simulink model "Simu_Simulink"  (R2016a)
settings: Solver=FixedStepDiscrete  StartTime=0.0  StopTime=50  FixedStep=0.01  RelTol=1e-3
values from neighbouring files (symbols this model uses):
  lambdaSplit = reshape(lambda,lambdaDim,sizeSeg,DoP)    [Simu_Matlab.m]    (also in Simu_Matlab_test.m = lambdaSplitNew; Simu_Simulink_Setup.m = reshape(lambda, lambdaDim,  sizeSeg,DoP))
  LAMBDASplit = reshape(LAMBDA,xDim,xDim,sizeSeg,DoP)    [Simu_Matlab.m]    (also in Simu_Matlab_test.m; Simu_Simulink_Setup.m = reshape(LAMBDA, xDim, xDim, sizeSeg,DoP))
  pSplit = reshape(par,pDim,sizeSeg,DoP)    [Simu_Matlab.m]    (also in Simu_Matlab_test.m; Simu_Simulink_Setup.m = reshape(par,    pDim,       sizeSeg,DoP))
  uSplit = reshape(u,uDim,sizeSeg,DoP)    [Simu_Matlab.m]    (also in Simu_Matlab_test.m; Simu_Simulink_Setup.m = reshape(u,      uDim,       sizeSeg,DoP))
  x0 = [1 0 1 0 1 0 0 0 0]    [GEN_initData.mat]    (also in NMPC_Problem_Formulation.m = [1;0;1;0;1;0;0;0;0]; Simu_Matlab.m = SIM_Plant_RK4(uOpt(1:4,1),x0,pSimVal,Ts); Simu_Matlab_test.m = SIM_Plant_RK4(uOpt(1:4,1),x0,pSimVal,Ts); Simu_Simulink_Setup.m = data.x0)
  xSplit = reshape(x,xDim,sizeSeg,DoP)    [Simu_Matlab.m]    (also in Simu_Matlab_test.m = xSplitNew; Simu_Simulink_Setup.m = reshape(x,      xDim,       sizeSeg,DoP))
settings Model: Creator=Deng  LastModifiedBy=Deng
settings OptimizationCC: SimCompilerOptimization=on
settings HardwareCC: ProdWordSize=32  ProdHWDeviceType=Specified
settings SFSimCC: SimCustomHeaderCode="#include \"NMPC_Iter.h\""  SimUserLibraries=NMPC_Iter.lib
settings SFSimCC: SimUserIncludeDirs=|
  | ./codegen/dll/NMPC_Iter
  | ./codegen/lib/OCP_F_Fu_Fx
settings RTWCC: GenerateReport=on  RTWUseSimCustomCode=on  CustomHeaderCode="#include \"NMPC_Iter.h\""  CustomLibrary=NMPC_Iter.lib  BuildConfiguration=Faster Runs  LaunchReport=on
settings RTWCC: CustomInclude=|
  | ./codegen/dll/NMPC_Iter
  | ./codegen/lib/OCP_F_Fu_Fx

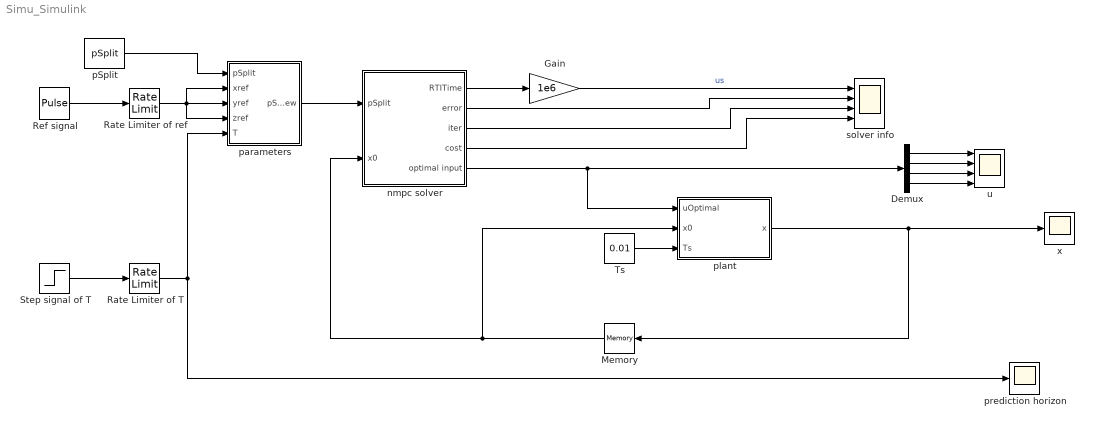
== system Simu_Simulink ==
  Demux : Demux
  Gain : Gain  Gain=1e6
  Memory : Memory  X0=x0
  Rate Limiter of T : RateLimiter  SampleTimeMode=inherited
  Rate Limiter of ref : RateLimiter  RisingSlewLimit=10  SampleTimeMode=inherited
  Ref signal : DiscretePulseGenerator  PulseType=Time based  Period=20  PulseWidth=50  PhaseDelay=10
  Step signal of T : Step  Time=25  Before=1  After=0.5  SampleTime=0
  Ts : Constant  Value=0.01
  nmpc solver : Subsystem
  pSplit : Constant  Value=pSplit
  parameters : MATLAB Function  TreatAsAtomicUnit=on
  plant : MATLAB Function  TreatAsAtomicUnit=on
  prediction horizon : Scope
  solver info : Scope  NumInputPorts=4
  u : Scope  NumInputPorts=4
  x : Scope
  wires:
  Memory/1 -> nmpc solver/2(x0), plant/2(x0)
  plant/1(x) -> Memory/1, x/1
  Ts/1 -> plant/3(Ts)
  pSplit/1 -> parameters/1(pSplit)
  Rate Limiter of ref/1 -> parameters/2(xref), parameters/4(zref), parameters/3(yref)
  parameters/1(pSplitNew) -> nmpc solver/1(pSplit)
  nmpc solver/5(optimal input) -> plant/1(uOptimal), Demux/1
  Demux/1 -> u/1
  Demux/2 -> u/2
  Demux/3 -> u/3
  Demux/4 -> u/4
  nmpc solver/2(error) -> solver info/2
  nmpc solver/1(RTITime) -> Gain/1
  nmpc solver/4(cost) -> solver info/4
  Ref signal/1 -> Rate Limiter of ref/1
  nmpc solver/3(iter) -> solver info/3
  Gain/1 -> solver info/1  "us"
  Step signal of T/1 -> Rate Limiter of T/1
  Rate Limiter of T/1 -> prediction horizon/1, parameters/5(T)

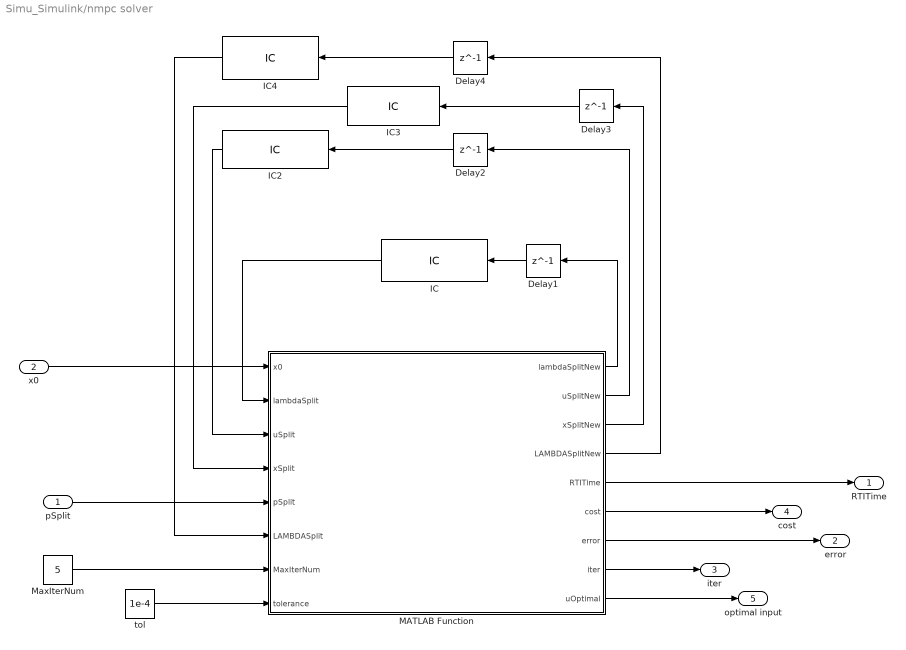
== system Simu_Simulink/nmpc solver ==
  pSplit : Inport
  x0 : Inport  Port=2
  Delay{1..4} (4 alike) : Delay  DelayLength=1  InitialCondition=0
  IC : InitialCondition  Value=lambdaSplit
  IC2 : InitialCondition  Value=uSplit
  IC3 : InitialCondition  Value=xSplit
  IC4 : InitialCondition  Value=LAMBDASplit
  MATLAB Function : MATLAB Function  TreatAsAtomicUnit=on
  MaxIterNum : Constant  Value=5
  tol : Constant  Value=1e-4
  RTITime : Outport
  error : Outport  Port=2
  iter : Outport  Port=3
  cost : Outport  Port=4
  optimal input : Outport  Port=5
  wires:
  Delay2/1 -> IC2/1
  Delay1/1 -> IC/1
  Delay4/1 -> IC4/1
  Delay3/1 -> IC3/1
  MaxIterNum/1 -> MATLAB Function/7(MaxIterNum)
  tol/1 -> MATLAB Function/8(tolerance)
  MATLAB Function/5(RTITime) -> RTITime/1
  MATLAB Function/6(cost) -> cost/1
  MATLAB Function/7(error) -> error/1
  MATLAB Function/9(uOptimal) -> optimal input/1
  x0/1 -> MATLAB Function/1(x0)
  MATLAB Function/8(iter) -> iter/1
  MATLAB Function/1(lambdaSplitNew) -> Delay1/1
  MATLAB Function/2(uSplitNew) -> Delay2/1
  MATLAB Function/3(xSplitNew) -> Delay3/1
  MATLAB Function/4(LAMBDASplitNew) -> Delay4/1
  IC/1 -> MATLAB Function/2(lambdaSplit)
  IC2/1 -> MATLAB Function/3(uSplit)
  IC3/1 -> MATLAB Function/4(xSplit)
  IC4/1 -> MATLAB Function/6(LAMBDASplit)
  pSplit/1 -> MATLAB Function/5(pSplit)

== matlab function Simu_Simulink/plant ==
  data: uOptimal input; x output; x0 input; Ts input
function x = plant(uOptimal,x0,Ts)
%#codegen
pSimVal = zeros(0,1);
x = SIM_Plant_RK4(uOptimal(:),x0,pSimVal,Ts);

== matlab function Simu_Simulink/nmpc solver/MATLAB Function ==
  data: lambdaSplitNew output; uSplitNew output; xSplitNew output; LAMBDASplitNew output; RTITime output; cost output; error output; iter output; uOptimal output; x0 input; lambdaSplit input; uSplit input; xSplit input; pSplit input; LAMBDASplit input; MaxIterNum input; tolerance input
function [lambdaSplitNew,uSplitNew, xSplitNew, LAMBDASplitNew,...
          RTITime, cost, error, iter, uOptimal] = ...
            nmpc_solver( x0,lambdaSplit,uSplit,...
                         xSplit,...
                         pSplit,...
                         LAMBDASplit,...
                         MaxIterNum,...
                         tolerance)
%#codegen
cost = 0;
error = 0;
timeElapsed = 0;
RTITime = 0;

coder.ceval('NMPC_Iter_initialize');
for iter=1:MaxIterNum
    % Executing in generated code, call C function 
    coder.ceval('NMPC_Iter',...
                 x0,...
                 coder.ref(lambdaSplit),...
                 coder.ref(uSplit),...
                 coder.ref(xSplit),...
                 coder.ref(pSplit),...
                 coder.ref(LAMBDASplit),...
                 coder.wref(cost),...
                 coder.wref(error),...
                 coder.wref(timeElapsed));
    RTITime = RTITime + timeElapsed;
    if error<tolerance
        break;
    end
end
lambdaSplitNew = lambdaSplit;
uSplitNew = uSplit;
xSplitNew = xSplit;
LAMBDASplitNew = LAMBDASplit;
uOptimal = uSplit(1:4,1,1);

== matlab function Simu_Simulink/parameters ==
  data: pSplit input; pSplitNew output; xref input; yref input; zref input; T input
function pSplitNew = fcn(pSplit,xref,yref,zref,T)
%#codegen
pSplitNew = pSplit;
pSplitNew(1,:,:) = xref;
pSplitNew(2,:,:) = yref;
pSplitNew(3,:,:) = zref;
pSplitNew(5,:,:) = T;
